simulink model "IMSPM_Q36121333_LAB2_SYSTEM"  (R2021b)
settings: Solver=VariableStepAuto  StartTime=0.0  StopTime=0.015  RelTol=1e-3
undefined symbols (not defined in the file or in its folder): plecs
settings Model: Creator=stanl  LastModifiedBy=stanl

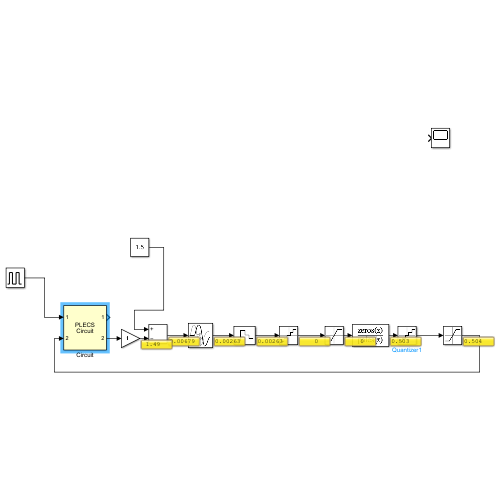
[thumbnail: Simulink's stored preview of the top-level diagram]
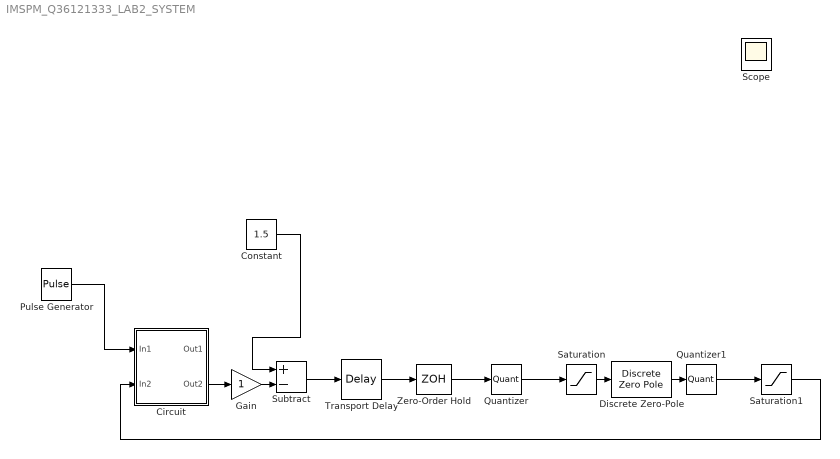
== system IMSPM_Q36121333_LAB2_SYSTEM ==
  Circuit : Subsystem  LoadFcn=plecs('sl', 200);  InitFcn=plecs('sl', 214);  StartFcn=plecs('sl', 208);  StopFcn=plecs('sl', 209);  mask(PlecsCircuit){PLECSData=<binary blob, 3548 chars, not shown>}
      mask prompts: PLECSData "PLECS Data (Do not delete or modify!)"
      mask init:
      | % PLACE CUSTOM INITIALIZATIONS ABOVE
      | % DO NOT REMOVE
      | plecs('sl', 215);
      | % DO NOT REMOVE
      settings: CopyFcn=plecs('sl', 203);  DeleteFcn=plecs('sl', 205);  UndoDeleteFcn=plecs('sl', 206);  PreSaveFcn=plecs('sl', 211);  PostSaveFcn=plecs('sl', 201);  NameChangeFcn=plecs('sl', 210);  DestroyFcn=plecs('sl', 207);  PreCopyFcn=plecs('sl', 216);  OpenFcn=plecs('sl', 202);  ErrorFcn=plerrorfcn
      mask Help: web(['file:///' fullfile(plecsdoc, 'creatingacircuit.html')])
      mask Display: disp('PLECS\nCircuit')
  Constant : Constant  Value=1.5
  Discrete Zero-Pole : DiscreteZeroPole  Zeros=[ 0.953 0.93]  Gain=5.8677  SampleTime=-1
  Gain : Gain
  Pulse Generator : DiscretePulseGenerator  PulseType=Time based  Amplitude=5  Period=0.004  PulseWidth=50  PhaseDelay=0.0002
  Quantizer : Quantizer  QuantizationInterval=0.0078125
  Quantizer1 : Quantizer  QuantizationInterval=0.001953125
  Saturation : Saturate  UpperLimit=0.03125  LowerLimit=-0.03125
  Saturation1 : Saturate  UpperLimit=0.95  LowerLimit=0.05
  Scope : Scope
  Subtract : Sum  Inputs=+-
  Transport Delay : TransportDelay  DelayTime=7e-7  InitialOutput=1.5  PadeOrder=5
  Zero-Order Hold : ZeroOrderHold  SampleTime=2e-6
  wires:
  Zero-Order Hold/1 -> Quantizer/1
  Saturation1/1 -> Circuit/2(In2)
  Circuit/2(Out2) -> Gain/1
  Subtract/1 -> Transport Delay/1
  Constant/1 -> Subtract/1
  Gain/1 -> Subtract/2
  Pulse Generator/1 -> Circuit/1(In1)
  Transport Delay/1 -> Zero-Order Hold/1
  Quantizer/1 -> Saturation/1
  Quantizer1/1 -> Saturation1/1
  Saturation/1 -> Discrete Zero-Pole/1
  Discrete Zero-Pole/1 -> Quantizer1/1

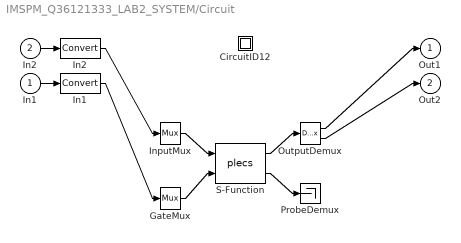
== system IMSPM_Q36121333_LAB2_SYSTEM/Circuit ==
  In1 : Inport  PortDimensions=1
  In2 : Inport  Port=2  PortDimensions=1
  " CircuitID12 " : Subsystem
  " GateMux " : Mux  Inputs=[ 1 ]
  " In1 " : DataTypeConversion  SaturateOnIntegerOverflow=on  RndMeth=Zero
  " In2 " : DataTypeConversion  SaturateOnIntegerOverflow=on  RndMeth=Zero
  " InputMux " : Mux  Inputs=[ 1 ]
  " OutputDemux " : Demux  Outputs=[ 1 1 ]
  " ProbeDemux " : Terminator
  " S-Function " : S-Function  FunctionName=plecs  SFunctionDeploymentMode=off  EnableBusSupport=off
  Out1 : Outport  PortDimensions=1
  Out2 : Outport  Port=2  PortDimensions=1
  wires:
  " InputMux "/1 -> " S-Function "/1
  " GateMux "/1 -> " S-Function "/2
  " S-Function "/1 -> " OutputDemux "/1
  " S-Function "/2 -> " ProbeDemux "/1
  In2/1 -> " In2 "/1
  " In2 "/1 -> " InputMux "/1
  In1/1 -> " In1 "/1
  " In1 "/1 -> " GateMux "/1
  " OutputDemux "/1 -> Out1/1
  " OutputDemux "/2 -> Out2/1

== system IMSPM_Q36121333_LAB2_SYSTEM/Circuit/ CircuitID12  ==
